simulink model "FINAL_A2"  (R2022b)
settings: Solver=FixedStepAuto  StartTime=0.0  StopTime=10.0  FixedStep=1e-3  RelTol=1e-3  EnableMultiTasking=on
undefined symbols (not defined in the file): A0, A1, D0, D1, D10, D11, D12, D13, D2, D3, D4, D5, D6, D7, D8, D9, magnitude, PTA0, PTA1, PTA2, PTB2, PTB23, PTB3, PTB9, PTC16, PTC17, PTC2, PTC3, PTC4, PTD0, PTD1, PTD2, PTD3
libraries: frdmk64flib x22, etargetslib x8
settings Model: ExtModeTrigDuration=5  Creator=sonja  LastModifiedBy=sonja
settings SolverCC: AlgebraicLoopSolver=TrustRegion
settings OptimizationCC: EnhancedBackFolding=on  PassReuseOutputArgsAs=Individual arguments  ZeroExternalMemoryAtStartup=off  ZeroInternalMemoryAtStartup=off  MaxStackSize=64  OptimizeBlockOrder=speed  DifferentSizesBufferReuse=on  OptimizationCustomize=off  EfficientTunableParamExpr=on
settings DebuggingCC: ParameterTunabilityLossMsg=error  UnconnectedInputMsg=warning  UnconnectedOutputMsg=warning  UnconnectedLineMsg=warning  SFMachineParentedDataDiag=warning
settings HardwareCC: ProdBitPerPointer=32  ProdBitPerSizeT=32  ProdBitPerPtrDiffT=32  ProdLargestAtomicInteger=Long  ProdLargestAtomicFloat=Double  ProdWordSize=32  ProdHWDeviceType=ARM Compatible->ARM Cortex
settings ModelReferenceCC: EnableRefExpFcnMdlSchedulingChecks=on
settings SFSimCC: MATLABDynamicMemAlloc=off
settings RTWCC: Description=Embedded Coder  SystemTargetFile=ert.tlc  HardwareBoard=NXP FRDM-K64F  TLCOptions="-aInlineSetEventsForThisBaseRateFcn=TLC_FALSE -aSuppressMultiTaskScheduler=TLC_FALSE  -aRateBasedStepFcn=0"  TemplateMakefile=ert_default_tmf  Toolchain=GNU Tools for ARM Embedded Processors  DLArmComputeVersion=19.05
settings CodeAppCC: ForceParamTrailComments=on  IgnoreCustomStorageClasses=off  OperatorAnnotations=on  SimulinkDataObjDesc=on  SFDataObjDesc=on  InsertBlockDesc=on
settings ERTTargetCC: ExtModeTransport=4  ExtModeMexFile=sendToCommService

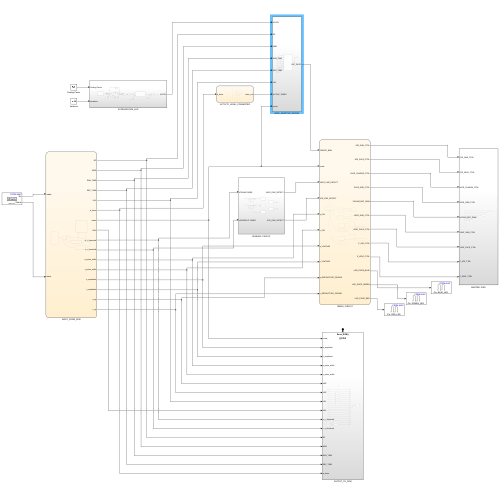
[thumbnail: Simulink's stored preview of the top-level diagram]
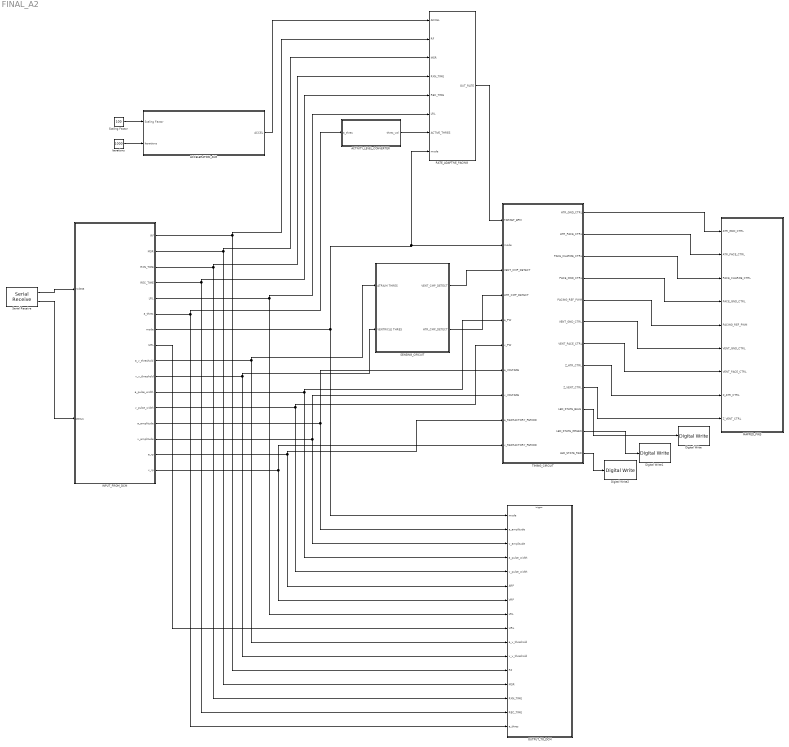
== system FINAL_A2 ==
  ACCELERATION_AVG : Subsystem
  ACTIVITY_LEVEL_CONVERTER : Stateflow chart  TreatAsAtomicUnit=on
  Digital Write : frdmk64flib/Digital Write  Whichpin=BLUE_LED
  Digital Write1 : frdmk64flib/Digital Write  Whichpin=GREEN_LED
  Digital Write2 : frdmk64flib/Digital Write  Whichpin=RED_LED
  INPUT_FROM_DCM : Stateflow chart  TreatAsAtomicUnit=on
      settings: PortSchema="{\"entries\":[{\"content\":{\"sides\":[{\"content\":{\"connectorIds\":[\"In1\",\"In2\"]},\"type\":\"ConnectorPlacement.EquallySpacedRectSide\",\"uuid\":\"325c6100-c23e-4e46-8539-863afd43e00a\"},{\"content\":{\"connectorIds\":[\"Out9\",\"Out10\",\"Out11\",\"Out13\",\"Out14\",\"Out12\",\"Out3\",\"Out15\",\"Out2\",\"Out1\",\"Out4\",\"Out5\",\"Out6\",\"Out7\",\"Out16\",\"Out8\"],\"side\":\"RIGHT\"},\"type\":\"ConnectorPlacement.EquallySpacedRectSide\",\"uuid\":\"9edcc76f-78cd-41fe-8bab-e11dd18f333e\"},{\"content\":{\"connectorIds\":[],\"side\":\"TOP\"},\"type\":\"ConnectorPlacement.EquallySpacedRectSide\",\"uuid\":\"22b5b9fd-d128-434d-acf7-bf8fc6cfb468\"}]},\"type\":\"ConnectorPlacement.EquallySpacedConnector\",\"uuid\":\"2a82357a-832c-4893-ba0c-363c88f62e72\"}],\"packageUris\":[\"http://schema.mathworks.com/mf0/Connector/R2020b\"],\"version\":\"1.0\"}"
  Iterations : Constant  Value=1000  OutDataTypeStr=single
  MAPPED_PINS : Subsystem
  OUTPUT_TO_DCM : Subsystem
  RATE_ADAPTIVE_PACING : Subsystem
  SENSING_CIRCUIT : Subsystem
  Scaling Factor : Constant  Value=100  OutDataTypeStr=single
  Serial Receive : frdmk64flib/Serial Receive  SCIModule=0  Baudrate=uint32(9600)  Parity=None  StopBits=1  HardwareFlowControl=None  ByteOrder=LittleEndian  DataType=uint8  DataLength=36  BlockingMode=off  OutputStatus=on  SampleTime=-1
  TIMING_CIRCUIT : Stateflow chart  TreatAsAtomicUnit=on
      settings: PortSchema="{\"entries\":[{\"content\":{\"sides\":[{\"content\":{\"connectorIds\":[\"In8\",\"In2\",\"In3\",\"In6\",\"In4\",\"In5\",\"In1\",\"In7\",\"In10\",\"In9\"]},\"type\":\"ConnectorPlacement.EquallySpacedRectSide\",\"uuid\":\"bc9f73e4-9637-4468-a4c1-5908944e8178\"},{\"content\":{\"connectorIds\":[\"Out1\",\"Out2\",\"Out3\",\"Out4\",\"Out5\",\"Out6\",\"Out7\",\"Out8\",\"Out9\",\"Out10\",\"Out11\",\"Out12\"],\"side\":\"RIGHT\"},\"type\":\"ConnectorPlacement.EquallySpacedRectSide\",\"uuid\":\"6b8161da-4ac1-4649-adbe-4e28d0f432d2\"},{\"content\":{\"connectorIds\":[],\"side\":\"TOP\"},\"type\":\"ConnectorPlacement.EquallySpacedRectSide\",\"uuid\":\"f9cafeb1-30dc-41ac-9268-fd8df2342768\"}]},\"type\":\"ConnectorPlacement.EquallySpacedConnector\",\"uuid\":\"2490419c-f1bb-4566-bca3-b4a855a26343\"}],\"packageUris\":[\"http://schema.mathworks.com/mf0/Connector/R2020b\"],\"version\":\"1.0\"}"
  wires:
  TIMING_CIRCUIT/1(ATR_GND_CTRL) -> MAPPED_PINS/1(ATR_GND_CTRL)
  TIMING_CIRCUIT/2(ATR_PACE_CTRL) -> MAPPED_PINS/2(ATR_PACE_CTRL)
  TIMING_CIRCUIT/3(PACE_CHARGE_CTRL) -> MAPPED_PINS/3(PACE_CHARGE_CTRL)
  TIMING_CIRCUIT/4(PACE_GND_CTRL) -> MAPPED_PINS/4(PACE_GND_CTRL)
  TIMING_CIRCUIT/5(PACING_REF_PWM) -> MAPPED_PINS/5(PACING_REF_PWM)
  TIMING_CIRCUIT/6(VENT_GND_CTRL) -> MAPPED_PINS/6(VENT_GND_CTRL)
  TIMING_CIRCUIT/7(VENT_PACE_CTRL) -> MAPPED_PINS/7(VENT_PACE_CTRL)
  TIMING_CIRCUIT/8(Z_ATR_CTRL) -> MAPPED_PINS/8(Z_ATR_CTRL)
  TIMING_CIRCUIT/9(Z_VENT_CTRL) -> MAPPED_PINS/9(Z_VENT_CTRL)
  TIMING_CIRCUIT/10(LED_STATE_BLUE) -> Digital Write/1
  TIMING_CIRCUIT/11(LED_STATE_GREEN) -> Digital Write1/1
  SENSING_CIRCUIT/1(VENT_CMP_DETECT) -> TIMING_CIRCUIT/3(VENT_CMP_DETECT)
  SENSING_CIRCUIT/2(ATR_CMP_DETECT) -> TIMING_CIRCUIT/6(ATR_CMP_DETECT)
  Serial Receive/1 -> INPUT_FROM_DCM/1(rxdata)
  Serial Receive/2 -> INPUT_FROM_DCM/2(status)
  INPUT_FROM_DCM/3(mode) -> TIMING_CIRCUIT/2(mode), RATE_ADAPTIVE_PACING/8(mode), OUTPUT_TO_DCM/1(mode)
  INPUT_FROM_DCM/4(a_pulse_width) -> TIMING_CIRCUIT/4(a_PW), OUTPUT_TO_DCM/4(a_pulse_width)
  INPUT_FROM_DCM/2(a_v_threshold) -> SENSING_CIRCUIT/1(ATRIUM THRES), OUTPUT_TO_DCM/10(a_v_threshold)
  INPUT_FROM_DCM/1(v_v_threshold) -> SENSING_CIRCUIT/2(VENTRICLE THRES), OUTPUT_TO_DCM/11(v_v_threshold)
  INPUT_FROM_DCM/5(v_pulse_width) -> TIMING_CIRCUIT/5(v_PW), OUTPUT_TO_DCM/5(v_pulse_width)
  ACCELERATION_AVG/1(ACCEL) -> RATE_ADAPTIVE_PACING/1(ACCEL)
  Scaling Factor/1 -> ACCELERATION_AVG/1("Scaling Factor ")
  Iterations/1 -> ACCELERATION_AVG/2(Iterations)
  ACTIVITY_LEVEL_CONVERTER/1(thres_val) -> RATE_ADAPTIVE_PACING/7(ACTIVE_THRES)
  INPUT_FROM_DCM/9(RF) -> RATE_ADAPTIVE_PACING/2(RF), OUTPUT_TO_DCM/12(RF)
  INPUT_FROM_DCM/10(MSR) -> RATE_ADAPTIVE_PACING/3(MSR), OUTPUT_TO_DCM/13(MSR)
  INPUT_FROM_DCM/11(RXN_TIME) -> RATE_ADAPTIVE_PACING/4(RXN_TIME), OUTPUT_TO_DCM/14(RXN_TIME)
  INPUT_FROM_DCM/13(REC_TIME) -> RATE_ADAPTIVE_PACING/5(REC_TIME), OUTPUT_TO_DCM/15(REC_TIME)
  INPUT_FROM_DCM/14(LRL) -> RATE_ADAPTIVE_PACING/6(LRL), OUTPUT_TO_DCM/8(LRL)
  INPUT_FROM_DCM/6(a_amplitude) -> TIMING_CIRCUIT/1(a_VOLTAGE), OUTPUT_TO_DCM/2(a_amplitude)
  INPUT_FROM_DCM/7(v_amplitude) -> TIMING_CIRCUIT/7(v_VOLTAGE), OUTPUT_TO_DCM/3(v_amplitude)
  INPUT_FROM_DCM/8(v_rp) -> TIMING_CIRCUIT/9(v_REFRACTORY_PERIOD), OUTPUT_TO_DCM/7(VRP)
  INPUT_FROM_DCM/12(a_thres) -> ACTIVITY_LEVEL_CONVERTER/1(a_thres), OUTPUT_TO_DCM/16(a_thres)
  INPUT_FROM_DCM/16(a_rp) -> TIMING_CIRCUIT/10(a_REFRACTORY_PERIOD), OUTPUT_TO_DCM/6(ARP)
  INPUT_FROM_DCM/15(URL) -> OUTPUT_TO_DCM/9(URL)
  TIMING_CIRCUIT/12(LED_STATE_RED) -> Digital Write2/1
  RATE_ADAPTIVE_PACING/1(OUT_RATE) -> TIMING_CIRCUIT/8(TARGET_BPM)

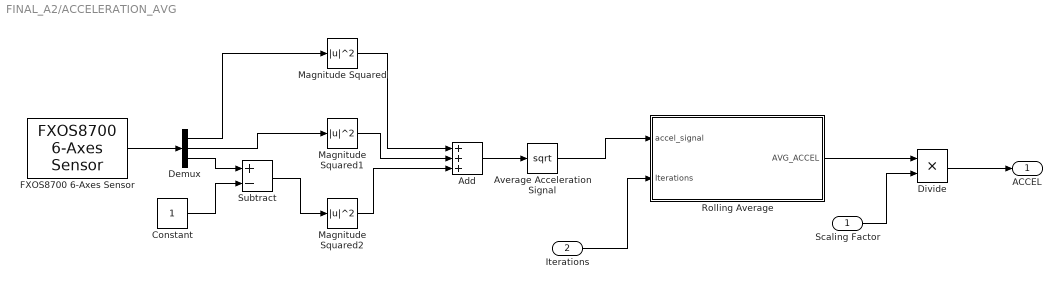
== system FINAL_A2/ACCELERATION_AVG ==
  "Scaling Factor " : Inport  OutDataTypeStr=single
  Iterations : Inport  Port=2  OutDataTypeStr=single
  Add : Sum  Inputs=+++  AccumDataTypeStr=single  OutDataTypeStr=single
  Average Acceleration Signal : Sqrt  OutDataTypeStr=single  IntermediateResultsDataTypeStr=single
  Constant : Constant  OutDataTypeStr=single
  Demux : Demux  Outputs=3
  Divide : Product  Inputs=**  OutDataTypeStr=single
  FXOS8700 6-Axes Sensor : frdmk64flib/FXOS8700 6-Axes Sensor  Activesensor=Accelerometer only  ODR=400Hz  HybridODR=400Hz  Accelfullrange=-4g to +4g  SampleTime=-1
  Magnitude Squared : Math  Operator=magnitude^2  OutDataTypeStr=single
  Magnitude Squared1 : Math  Operator=magnitude^2  OutDataTypeStr=single
  Magnitude Squared2 : Math  Operator=magnitude^2  OutDataTypeStr=single
  Rolling Average : Stateflow chart  TreatAsAtomicUnit=on
  Subtract : Sum  Inputs=+-  AccumDataTypeStr=single  OutDataTypeStr=single
  ACCEL : Outport  OutDataTypeStr=single
  wires:
  Demux/2 -> Magnitude Squared1/1
  Magnitude Squared1/1 -> Add/2
  Magnitude Squared/1 -> Add/1
  Demux/1 -> Magnitude Squared/1
  Demux/3 -> Subtract/1
  Magnitude Squared2/1 -> Add/3
  Subtract/1 -> Magnitude Squared2/1
  Constant/1 -> Subtract/2
  FXOS8700 6-Axes Sensor/1 -> Demux/1
  Add/1 -> Average Acceleration Signal/1
  Average Acceleration Signal/1 -> Rolling Average/1(accel_signal)
  Rolling Average/1(AVG_ACCEL) -> Divide/1
  "Scaling Factor "/1 -> Divide/2
  Divide/1 -> ACCEL/1
  Iterations/1 -> Rolling Average/2(Iterations)

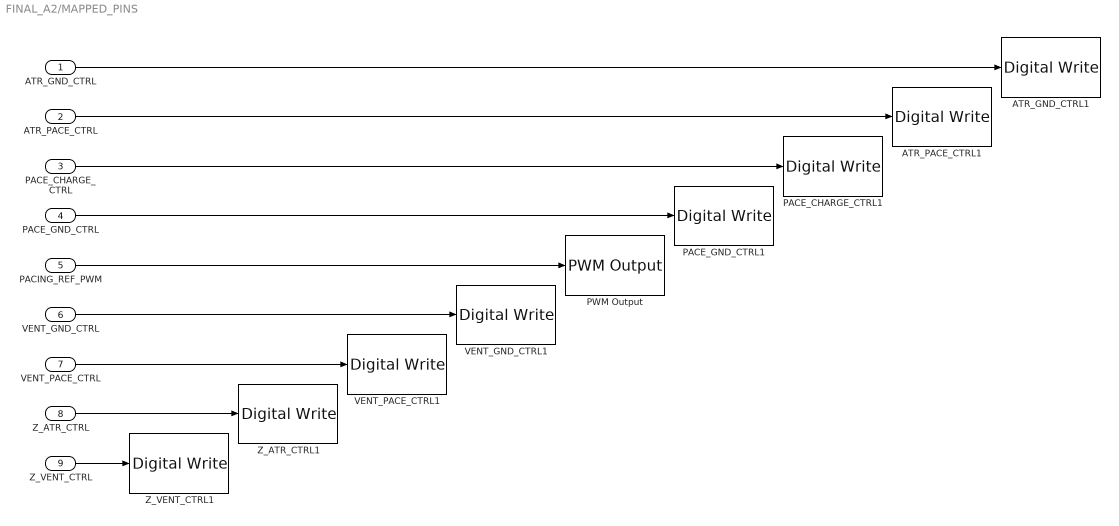
== system FINAL_A2/MAPPED_PINS ==
  ATR_GND_CTRL : Inport
  ATR_PACE_CTRL : Inport  Port=2
  PACE_CHARGE_CTRL : Inport  Port=3
  PACE_GND_CTRL : Inport  Port=4
  PACING_REF_PWM : Inport  Port=5
  VENT_GND_CTRL : Inport  Port=6
  VENT_PACE_CTRL : Inport  Port=7
  Z_ATR_CTRL : Inport  Port=8
  Z_VENT_CTRL : Inport  Port=9
  ATR_GND_CTRL1 : frdmk64flib/Digital Write  Whichpin=PTD2 (D11)
  ATR_PACE_CTRL1 : frdmk64flib/Digital Write  Whichpin=PTA0 (D8)
  PACE_CHARGE_CTRL1 : frdmk64flib/Digital Write  Whichpin=PTB9 (D2)
  PACE_GND_CTRL1 : frdmk64flib/Digital Write  Whichpin=PTD0 (D10)
  PWM Output : frdmk64flib/PWM Output  Whichpin=PTA2 (D5)  InitialFrequency=2000  InitialDutyCycle=0
  VENT_GND_CTRL1 : frdmk64flib/Digital Write  Whichpin=PTD3 (D12)
  VENT_PACE_CTRL1 : frdmk64flib/Digital Write  Whichpin=PTC4 (D9)
  Z_ATR_CTRL1 : frdmk64flib/Digital Write  Whichpin=PTB23 (D4)
  Z_VENT_CTRL1 : frdmk64flib/Digital Write  Whichpin=PTC3 (D7)
  wires:
  ATR_GND_CTRL/1 -> ATR_GND_CTRL1/1
  ATR_PACE_CTRL/1 -> ATR_PACE_CTRL1/1
  PACE_CHARGE_CTRL/1 -> PACE_CHARGE_CTRL1/1
  PACE_GND_CTRL/1 -> PACE_GND_CTRL1/1
  PACING_REF_PWM/1 -> PWM Output/1
  VENT_GND_CTRL/1 -> VENT_GND_CTRL1/1
  VENT_PACE_CTRL/1 -> VENT_PACE_CTRL1/1
  Z_ATR_CTRL/1 -> Z_ATR_CTRL1/1
  Z_VENT_CTRL/1 -> Z_VENT_CTRL1/1

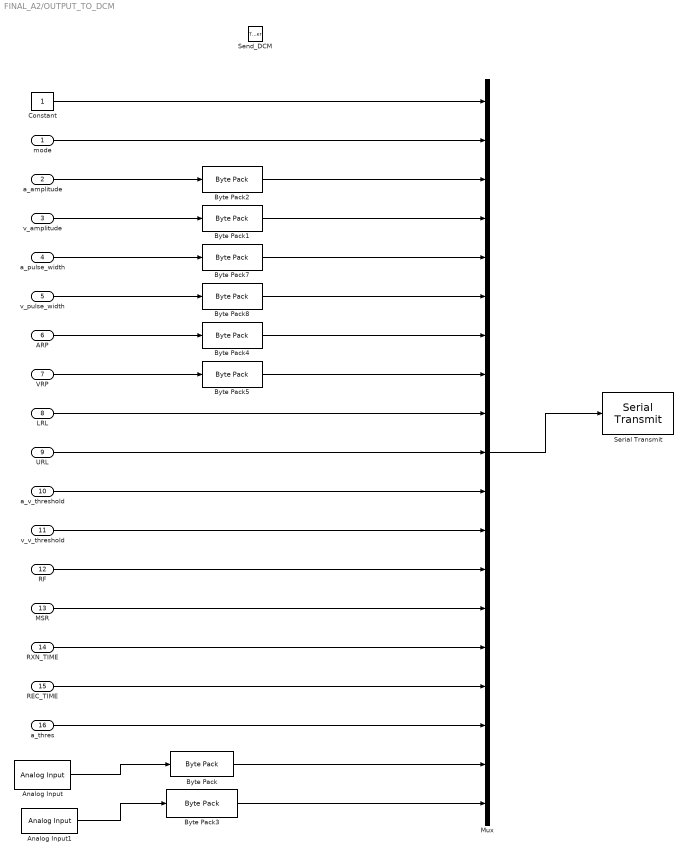
== system FINAL_A2/OUTPUT_TO_DCM ==
  mode : Inport  OutDataTypeStr=uint8
  a_amplitude : Inport  Port=2  OutDataTypeStr=double
  v_amplitude : Inport  Port=3  OutDataTypeStr=double
  a_pulse_width : Inport  Port=4  OutDataTypeStr=uint16
  v_pulse_width : Inport  Port=5  OutDataTypeStr=uint16
  ARP : Inport  Port=6  OutDataTypeStr=uint16
  VRP : Inport  Port=7  OutDataTypeStr=uint16
  LRL : Inport  Port=8  OutDataTypeStr=uint8
  URL : Inport  Port=9
  a_v_threshold : Inport  Port=10  OutDataTypeStr=uint8
  v_v_threshold : Inport  Port=11  OutDataTypeStr=uint8
  RF : Inport  Port=12  OutDataTypeStr=uint8
  MSR : Inport  Port=13  OutDataTypeStr=uint8
  RXN_TIME : Inport  Port=14  OutDataTypeStr=uint8
  REC_TIME : Inport  Port=15  OutDataTypeStr=uint8
  a_thres : Inport  Port=16  OutDataTypeStr=uint8
  Send_DCM : TriggerPort  TriggerType=function-call  IsSimulinkFunction=on  FunctionName=Send_DCM  VariantControl=Variant
  Analog Input : frdmk64flib/Analog Input  Whichpin=PTB2 (A0)  SampleTime=-1
  Analog Input1 : frdmk64flib/Analog Input  Whichpin=PTB3 (A1)  SampleTime=-1
  Byte Pack{,1..3} (4 alike) : etargetslib/Byte Pack  datatypes={'double'}  byteAlign=1
  Byte Pack{4..5,7..8} (4 alike) : etargetslib/Byte Pack  datatypes={'uint16'}  byteAlign=1
  Constant : Constant  OutDataTypeStr=uint8
  Mux : Mux  Inputs=19
  Serial Transmit : frdmk64flib/Serial Transmit  SCIModule=0  Baudrate=uint32(9600)  Parity=None  StopBits=1  HardwareFlowControl=None  ByteOrder=LittleEndian  BlockingMode=on  OutputStatus=off
  wires:
  v_amplitude/1 -> Byte Pack1/1
  a_amplitude/1 -> Byte Pack2/1
  VRP/1 -> Byte Pack5/1
  ARP/1 -> Byte Pack4/1
  v_pulse_width/1 -> Byte Pack8/1
  a_pulse_width/1 -> Byte Pack7/1
  Constant/1 -> Mux/1
  mode/1 -> Mux/2
  Byte Pack1/1 -> Mux/4
  Byte Pack2/1 -> Mux/3
  Byte Pack7/1 -> Mux/5
  Byte Pack8/1 -> Mux/6
  Mux/1 -> Serial Transmit/1
  Byte Pack4/1 -> Mux/7
  Byte Pack5/1 -> Mux/8
  LRL/1 -> Mux/9
  URL/1 -> Mux/10
  a_v_threshold/1 -> Mux/11
  v_v_threshold/1 -> Mux/12
  RF/1 -> Mux/13
  MSR/1 -> Mux/14
  RXN_TIME/1 -> Mux/15
  REC_TIME/1 -> Mux/16
  a_thres/1 -> Mux/17
  Analog Input/1 -> Byte Pack/1
  Analog Input1/1 -> Byte Pack3/1
  Byte Pack/1 -> Mux/18
  Byte Pack3/1 -> Mux/19

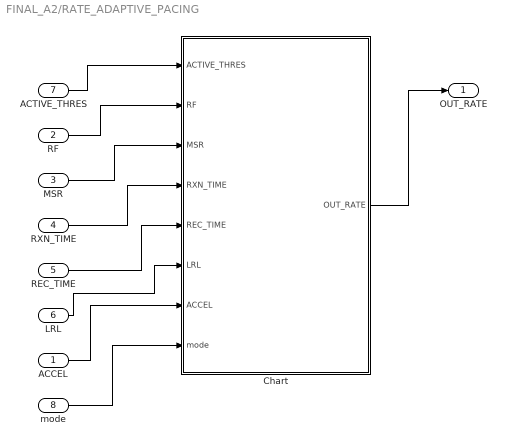
== system FINAL_A2/RATE_ADAPTIVE_PACING ==
  ACCEL : Inport  OutDataTypeStr=single
  RF : Inport  Port=2  OutDataTypeStr=uint8
  MSR : Inport  Port=3  OutDataTypeStr=uint8
  RXN_TIME : Inport  Port=4  OutDataTypeStr=uint8
  REC_TIME : Inport  Port=5  OutDataTypeStr=uint8
  LRL : Inport  Port=6  OutDataTypeStr=uint8
  ACTIVE_THRES : Inport  Port=7  OutDataTypeStr=single
  mode : Inport  Port=8  OutDataTypeStr=uint8
  Chart : Stateflow chart  TreatAsAtomicUnit=on
  OUT_RATE : Outport  OutDataTypeStr=double
  wires:
  ACTIVE_THRES/1 -> Chart/1(ACTIVE_THRES)
  RF/1 -> Chart/2(RF)
  MSR/1 -> Chart/3(MSR)
  RXN_TIME/1 -> Chart/4(RXN_TIME)
  REC_TIME/1 -> Chart/5(REC_TIME)
  LRL/1 -> Chart/6(LRL)
  ACCEL/1 -> Chart/7(ACCEL)
  Chart/1(OUT_RATE) -> OUT_RATE/1
  mode/1 -> Chart/8(mode)

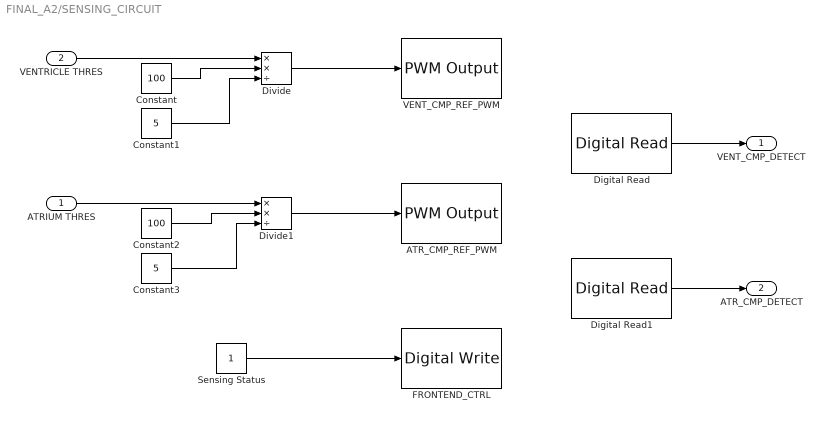
== system FINAL_A2/SENSING_CIRCUIT ==
  ATRIUM THRES : Inport  OutDataTypeStr=uint8
  VENTRICLE THRES : Inport  Port=2  OutDataTypeStr=uint8
  ATR_CMP_REF_PWM : frdmk64flib/PWM Output  Whichpin=PTC2 (D6)  InitialFrequency=2000  InitialDutyCycle=0
  Constant : Constant  Value=100  OutDataTypeStr=uint8
  Constant1 : Constant  Value=5  OutDataTypeStr=uint8
  Constant2 : Constant  Value=100  OutDataTypeStr=uint8
  Constant3 : Constant  Value=5  OutDataTypeStr=uint8
  Digital Read : frdmk64flib/Digital Read  Whichpin=PTC17 (D1)  SampleTime=-1
  Digital Read1 : frdmk64flib/Digital Read  Whichpin=PTC16 (D0)  SampleTime=-1
  Divide : Product  Inputs=**/  OutDataTypeStr=single
  Divide1 : Product  Inputs=**/  OutDataTypeStr=single
  FRONTEND_CTRL : frdmk64flib/Digital Write  Whichpin=PTD1 (D13)
  Sensing Status : Constant  OutDataTypeStr=uint8
  VENT_CMP_REF_PWM : frdmk64flib/PWM Output  Whichpin=PTA1 (D3)  InitialFrequency=2000  InitialDutyCycle=0
  VENT_CMP_DETECT : Outport  OutDataTypeStr=boolean
  ATR_CMP_DETECT : Outport  Port=2  OutDataTypeStr=boolean
  wires:
  ATRIUM THRES/1 -> Divide1/1
  Constant/1 -> Divide/2
  VENTRICLE THRES/1 -> Divide/1
  Constant1/1 -> Divide/3
  Constant2/1 -> Divide1/2
  Constant3/1 -> Divide1/3
  Divide/1 -> VENT_CMP_REF_PWM/1
  Divide1/1 -> ATR_CMP_REF_PWM/1
  Digital Read1/1 -> ATR_CMP_DETECT/1
  Digital Read/1 -> VENT_CMP_DETECT/1
  Sensing Status/1 -> FRONTEND_CTRL/1

== stateflow chart FINAL_A2/ACCELERATION_AVG/Rolling Average ==
  state Setting_Var
    entry:
    count = 0;
    avg_signal = 0;
  state Accumulate_Signal
    entry:
    avg_signal = avg_signal + accel_signal;
    count = count + 1;
  state Average_Signal
    entry:
    avg_signal = avg_signal/count;
    AVG_ACCEL = avg_signal;
  (default) -> Setting_Var
  Average_Signal -> Setting_Var
  Setting_Var -> Accumulate_Signal
  Accumulate_Signal -> Average_Signal [order 1] : [count >= Iterations]
  Accumulate_Signal -> Accumulate_Signal [order 2] : [count < Iterations]
  data: accel_signal input single; AVG_ACCEL output single; Iterations input single; avg_signal local single; count local single

== stateflow chart FINAL_A2/INPUT_FROM_DCM ==
  settings: executeAtInitialization=1
  state SET_PARAMATERS
    entry:
    mode = uint8(rxdata(3));
    a_amplitude = typecast(rxdata(4:11), 'double');
    v_amplitude = typecast(rxdata(12:19), 'double')
    a_pulse_width = typecast(rxdata(20:21), 'uint16');
    v_pulse_width = typecast(rxdata(22:23), 'uint16');
    a_rp = typecast(rxdata(24:25), 'uint16');
    v_rp = typecast(rxdata(26:27), 'uint16');
    LRL = uint8(rxdata(28));
    URL = uint8(rxdata(29));
    %sensitivities
    a_v_threshold = uint8(rxdata(30));
    v_v_threshold = uint8(rxdata(31));
    %rate pacing
    RF = uint8(rxdata(32));
    MSR = uint8(rxdata(33));
    RXN_TIME = uint8(rxdata(34));
    REC_TIME = uint8(rxdata(35));
    a_thres = uint8(rxdata(36));
  state INITIAL_PARAMETERS
    entry:
    %default values here
    mode = uint8(1);
    a_pulse_width = uint16(1);
    v_pulse_width = uint16(1);
    a_amplitude = 50;
    v_amplitude = 50;
    a_rp = uint16(250);
    v_rp = uint16(320);
    LRL = uint8(60); %in bpm
    URL = uint8(120); %in bpm
    %sensitivities:
    v_v_threshold = uint8(3);
    a_v_threshold = uint8(3);
    %rate pacing
    RF = uint8(8);
    MSR = uint8(180);
    RXN_TIME = uint8(30);
    REC_TIME = uint8(10);
    a_thres = uint8(3);
  state STANDBY
    %waiting for DCM
  state ECHO_EGRAM
    entry:
    Send_DCM();
  state ECHO_PARAMATERS
    entry:
    Send_DCM();
  (default) -> INITIAL_PARAMETERS
  (junction 8) -> SET_PARAMATERS [order 1] : [rxdata(2) == hex2dec('55')]
  SET_PARAMATERS -> ECHO_EGRAM
  (junction 7) -> STANDBY [order 2]
  INITIAL_PARAMETERS -> STANDBY
  STANDBY -> (junction 7) : [status == 0]
  (junction 7) -> (junction 8) [order 1] : [rxdata(1) == hex2dec('16')]
  (junction 8) -> ECHO_PARAMATERS [order 2] : [rxdata(2) == hex2dec('22')]
  ECHO_PARAMATERS -> STANDBY
  ECHO_EGRAM -> STANDBY
  data: v_v_threshold output uint8; a_v_threshold output uint8; rxdata input uint8; status input uint8; mode output uint8; a_pulse_width output uint16; v_pulse_width output uint16; a_amplitude output double; v_amplitude output double; v_rp output uint16; RF output uint8; MSR output uint8; RXN_TIME output uint8; a_thres output uint8; REC_TIME output uint8; LRL output uint8; URL output; a_rp output uint16

== stateflow chart FINAL_A2/TIMING_CIRCUIT ==
  state Main
    entry:
    %where variables are set for hardware hiding
    %typecast(TARGET_BPM, 'uint16');
    LRI =double(60000./TARGET_BPM);
    typecast(a_PW, 'uint16');
    typecast(v_PW, 'uint16');
    %read as uint8 from dcm to save space
    %, then converted to uint16 for interactions between uint16s
    LED_STATE_RED = true;
  state CHARGING_C22_VENTRICLE
    entry:
    LED_STATE_GREEN = true;
    LED_STATE_BLUE = false;
    PACE_CHARGE_CTRL = true;
    PACE_GND_CTRL = true;
    VENT_PACE_CTRL = false;
    Z_ATR_CTRL = false;
    Z_VENT_CTRL = false;
    ATR_PACE_CTRL = false;
    VENT_GND_CTRL = true;
    PACING_REF_PWM = v_VOLTAGE;
  state DISCHARGE_C22_VENTRICLE
    entry:
    LED_STATE_GREEN = false;
    LED_STATE_BLUE = true;
    PACE_GND_CTRL = true;
    VENT_PACE_CTRL = true;
    Z_ATR_CTRL = false;
    Z_VENT_CTRL = false;
    ATR_PACE_CTRL = false;
    ATR_GND_CTRL = false;
    VENT_GND_CTRL = false;
  state CHARGING_C22_ATRIUM
    entry:
    LED_STATE_GREEN = true;
    LED_STATE_BLUE = false;
    PACE_CHARGE_CTRL = true;
    PACE_GND_CTRL = true;
    VENT_PACE_CTRL = false;
    Z_ATR_CTRL = false;
    Z_VENT_CTRL = false;
    ATR_PACE_CTRL = false;
    VENT_GND_CTRL = false;
    ATR_GND_CTRL = true;
    PACING_REF_PWM = a_VOLTAGE;
  state DISCHARGE_C22_ATRIUM
    entry:
    LED_STATE_GREEN = false;
    LED_STATE_BLUE = true;
    PACE_GND_CTRL = true;
    VENT_PACE_CTRL = false;
    Z_ATR_CTRL = false;
    Z_VENT_CTRL = false;
    ATR_PACE_CTRL = true;
    ATR_GND_CTRL = false;
    VENT_GND_CTRL = false;
  state DISCHARGING
    entry:
    LED_STATE_GREEN = false;
    LED_STATE_BLUE = true;
    PACE_GND_CTRL = true;
    VENT_PACE_CTRL = true;
    Z_ATR_CTRL = false;
    Z_VENT_CTRL = false;
    ATR_PACE_CTRL = false;
    ATR_GND_CTRL = false;
    VENT_GND_CTRL = false;
  state CHARGING1
    entry:
    LED_STATE_GREEN = true;
    LED_STATE_BLUE = false;
    PACE_CHARGE_CTRL = true;
    PACE_GND_CTRL = true;
    VENT_PACE_CTRL = false;
    Z_ATR_CTRL = false;
    Z_VENT_CTRL = false;
    ATR_PACE_CTRL = false;
    VENT_GND_CTRL = true;
    PACING_REF_PWM = v_VOLTAGE;
  state SENSING3
    %LRI=LRI- double(v_PW);
    REFRACT_PERIOD = v_REFRACTORY_PERIOD - v_PW;
  state SENSING
    REFRACT_PERIOD = v_REFRACTORY_PERIOD;
    LRI=double(60000./TARGET_BPM);
  state DISCHARGE_C22_ATRIUM1
    entry:
    LED_STATE_GREEN = false;
    LED_STATE_BLUE = true;
    PACE_GND_CTRL = true;
    VENT_PACE_CTRL = false;
    Z_ATR_CTRL = false;
    Z_VENT_CTRL = false;
    ATR_PACE_CTRL = true;
    ATR_GND_CTRL = false;
    VENT_GND_CTRL = false;
  state CHARGING_C22_ATRIUM1
    entry:
    LED_STATE_GREEN = true;
    LED_STATE_BLUE = false;
    PACE_CHARGE_CTRL = true;
    PACE_GND_CTRL = true;
    VENT_PACE_CTRL = false;
    Z_ATR_CTRL = false;
    Z_VENT_CTRL = false;
    ATR_PACE_CTRL = false;
    VENT_GND_CTRL = false;
    ATR_GND_CTRL = true;
    PACING_REF_PWM = a_VOLTAGE;
  state SENSING2
    %LRI=LRI-double(a_PW);
    REFRACT_PERIOD = a_REFRACTORY_PERIOD - a_PW;
  state SENSING1
    REFRACT_PERIOD = a_REFRACTORY_PERIOD;
    LRI=double(60000./TARGET_BPM);
  (default) -> Main
  CHARGING_C22_VENTRICLE -> DISCHARGE_C22_VENTRICLE : after(LRI - double(v_PW),msec)
  Main -> CHARGING_C22_VENTRICLE [order 1] : [mode == 1] %VOO
  Main -> SENSING1 [order 4] : after(a_REFRACTORY_PERIOD,msec)[mode==4] %AAI
  Main -> SENSING [order 3] : after(v_REFRACTORY_PERIOD,msec)[mode == 3] %VVI
  Main -> CHARGING_C22_ATRIUM [order 2] : [mode == 2] %AOO
  DISCHARGE_C22_VENTRICLE -> CHARGING_C22_VENTRICLE : after(v_PW,msec)
  CHARGING_C22_ATRIUM -> DISCHARGE_C22_ATRIUM : after(LRI-double(a_PW),msec)
  DISCHARGE_C22_ATRIUM -> CHARGING_C22_ATRIUM : after(a_PW,msec)
  CHARGING1 -> DISCHARGING [order 1] : after(LRI-double(v_PW),msec)
  DISCHARGING -> SENSING3 : after(v_PW,msec)
  SENSING3 -> CHARGING1
  SENSING -> CHARGING1
  CHARGING1 -> SENSING [order 2] : after(REFRACT_PERIOD,msec)[VENT_CMP_DETECT == true]
  CHARGING_C22_ATRIUM1 -> DISCHARGE_C22_ATRIUM1 [order 1] : after(LRI-double(a_PW),msec)
  DISCHARGE_C22_ATRIUM1 -> SENSING2 : after(a_PW,msec)
  SENSING2 -> CHARGING_C22_ATRIUM1
  SENSING1 -> CHARGING_C22_ATRIUM1
  CHARGING_C22_ATRIUM1 -> SENSING1 [order 2] : after(REFRACT_PERIOD,msec)[ATR_CMP_DETECT==true]
  data: ATR_GND_CTRL output boolean; ATR_PACE_CTRL output boolean; PACE_CHARGE_CTRL output boolean; PACE_GND_CTRL output boolean; PACING_REF_PWM output double; VENT_GND_CTRL output boolean; VENT_PACE_CTRL output boolean; a_VOLTAGE input double; mode input uint8; Z_ATR_CTRL output boolean; Z_VENT_CTRL output boolean; LED_STATE_BLUE output boolean; LED_STATE_GREEN output boolean; VENT_CMP_DETECT input boolean; a_PW input uint16; v_PW input uint16; ATR_CMP_DETECT input boolean; v_VOLTAGE input double; TARGET_BPM input double; v_REFRACTORY_PERIOD input uint16; LRI local double; a_REFRACTORY_PERIOD input uint16; REFRACT_PERIOD local uint16; LED_STATE_RED output boolean

== stateflow chart FINAL_A2/ACTIVITY_LEVEL_CONVERTER ==
  state V_Low_Threshold
    entry:
    thres_val = 20;
  state Low_Threshold
    entry:
    thres_val = 40;
  state EXIT1
  state Med_Low_Threshold
    entry:
    thres_val = 60;
  state Med_Threshold
    entry:
    thres_val = 80;
  state Med_High_Threshold
    entry:
    thres_val = 100;
  state High_Threshold
    entry:
    thres_val = 120;
  state EXIT2
  state V_High_Threshold
    entry:
    thres_val = 150;
  EXIT1 -> (junction 8)
  (default) -> (junction 8)
  V_Low_Threshold -> EXIT1
  EXIT2 -> (junction 8)
  (junction 8) -> V_Low_Threshold [order 1] : [a_thres == ActivityLevel.V_Low ]
  (junction 8) -> (junction 10) [order 2]
  (junction 10) -> Low_Threshold [order 1] : [a_thres == ActivityLevel.Low]
  Low_Threshold -> EXIT1
  (junction 10) -> (junction 17) [order 2]
  Med_Low_Threshold -> EXIT1
  Med_Threshold -> EXIT1
  Med_High_Threshold -> EXIT1
  V_High_Threshold -> EXIT1
  High_Threshold -> EXIT1
  (junction 17) -> Med_Low_Threshold [order 1] : [a_thres == ActivityLevel.Med_Low]
  (junction 17) -> (junction 21) [order 2]
  (junction 21) -> Med_Threshold [order 1] : [a_thres == ActivityLevel.Med]
  (junction 21) -> (junction 24) [order 2]
  (junction 24) -> Med_High_Threshold [order 1] : [a_thres == ActivityLevel.Med_High]
  (junction 24) -> (junction 28) [order 2]
  (junction 28) -> High_Threshold [order 1] : [a_thres == ActivityLevel.High]
  (junction 28) -> (junction 32) [order 2]
  (junction 32) -> EXIT2 [order 2]
  (junction 32) -> V_High_Threshold [order 1] : [a_thres == ActivityLevel.V_High]
  data: a_thres input uint8; thres_val output single

== stateflow chart FINAL_A2/RATE_ADAPTIVE_PACING/Chart ==
  state OUTPUT_RATE
    entry:
    %typecast(OUT_RATE,'double');
    OUT_RATE = double(NEW_RATE);
  state RATE_CALC
    entry:
    %converted to ms
    RATE_INC = (single(MSR)-single(LRL))/(1000*single(RXN_TIME));
    RATE_DEC = (single(MSR)-single(LRL))/(60000*single(REC_TIME));
  state MODE
  state SLOPE_CALC
    entry:
    slope = single(RF/10);
    GOAL_RATE = slope*(single(ACCEL)-single(ACTIVE_THRES)) + single(LRL);
  state INIT_STATE
  state LESS_THAN_LRL
    entry:
    GOAL_RATE = single(LRL);
  state SET_LRL
    entry:
    % if in any of the modes
    NEW_RATE = single(LRL);
  state GREATER_THAN_MSR
    entry:
    GOAL_RATE = single(MSR);
  state REACTION_TIME_RATE
    entry:
    NEW_RATE = NEW_RATE + 100*RATE_INC;
  state RECOVERY_TIME_RATE
    entry:
    NEW_RATE = NEW_RATE - 100*RATE_DEC;
  OUTPUT_RATE -> INIT_STATE : after(100,msec)
  MODE -> OUTPUT_RATE [order 2]
  SLOPE_CALC -> RATE_CALC [order 3]
  LESS_THAN_LRL -> RATE_CALC
  (default) -> INIT_STATE
  REACTION_TIME_RATE -> MODE
  RATE_CALC -> MODE [order 3]
  GREATER_THAN_MSR -> RATE_CALC
  RECOVERY_TIME_RATE -> MODE
  MODE -> SET_LRL [order 1] : [mode == 1 || mode == 2 || mode == 3 || mode == 4]
  SET_LRL -> MODE
  INIT_STATE -> SLOPE_CALC : {NEW_RATE = single(LRL)}
  SLOPE_CALC -> GREATER_THAN_MSR [order 1] : [GOAL_RATE>MSR]
  SLOPE_CALC -> LESS_THAN_LRL [order 2] : [GOAL_RATE < LRL]
  RATE_CALC -> REACTION_TIME_RATE [order 1] : [NEW_RATE < GOAL_RATE]
  RATE_CALC -> RECOVERY_TIME_RATE [order 2] : [NEW_RATE > GOAL_RATE]
  data: ACTIVE_THRES input single; RF input uint8; MSR input uint8; RXN_TIME input uint8; REC_TIME input uint8; LRL input uint8; ACCEL input single; slope local single; GOAL_RATE local single; OUT_RATE output double; RATE_DEC local single; NEW_RATE local single; RATE_INC local single; mode input uint8
